simulink model "Modulation"  (Simulink 6.0)
settings: Solver=ode45  StartTime=0.0  StopTime=10.0  RelTol=1e-3
settings Model: LastModifiedBy=arekg
settings DataIOCC: SignalLoggingName=sigsOut
settings DebuggingCC: SolverPrmCheckMsg=none
settings HardwareCC: TargetUnknown=on
settings GRTTargetCC: ModelReferenceCompliant=off  MatFileLogging=off

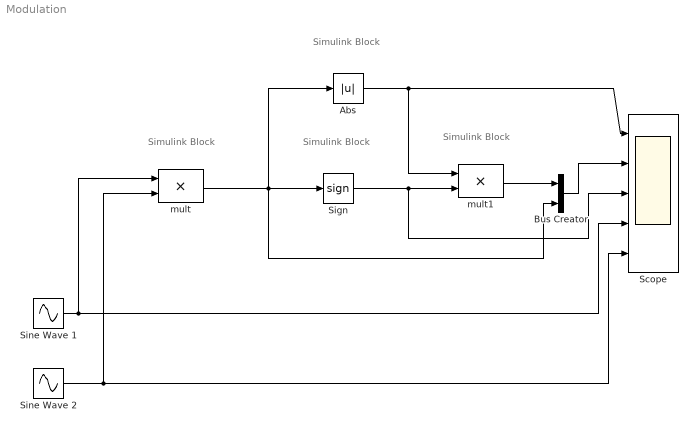
== system Modulation ==
  note: Simulink Block
  note: Simulink Block
  note: Simulink Block
  note: Simulink Block
  Abs : Abs  ZeroCross=off  SaturateOnIntegerOverflow=on
  Bus Creator : BusCreator  DialogController=Simulink.DDGSource_Bus  Inputs=2
  Scope : Scope  NumInputPorts=5
      settings: YMin=-1~-40~-2~-1~-1.5  YMax=40~40~2~40~1.5
  Sign : Signum  ZeroCross=off
  Sine Wave 1 : Sin  Amplitude=18  Bias=20  Frequency=0.5*pi  Phase=pi/1.3  SampleTime=1/10
  Sine Wave 2 : Sin  Amplitude=0.9  Frequency=pi/0.4  Phase=pi  SampleTime=1/20
  mult : Product  OutDataTypeMode=double  SaturateOnIntegerOverflow=on  RndMeth=Zero
  mult1 : Product  SaturateOnIntegerOverflow=on
  wires:
  Abs/1 -> mult1/1, Scope/1
  Sine Wave 1/1 -> Scope/4, mult/1
  Sine Wave 2/1 -> Scope/5, mult/2
  mult/1 -> Abs/1, Sign/1, Bus Creator/2
  Sign/1 -> mult1/2, Scope/3
  mult1/1 -> Bus Creator/1
  Bus Creator/1 -> Scope/2
